simulink model "databydata"  (R2024a)
settings: Solver=FixedStepAuto  StartTime=0.0  StopTime=1  FixedStep=0.01  RelTol=1e-3
libraries: simulink x1
settings Model: Creator=wsl  LastModifiedBy=wsl

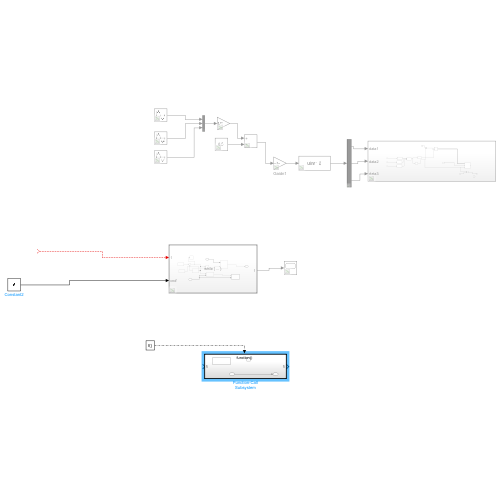
[thumbnail: Simulink's stored preview of the top-level diagram]
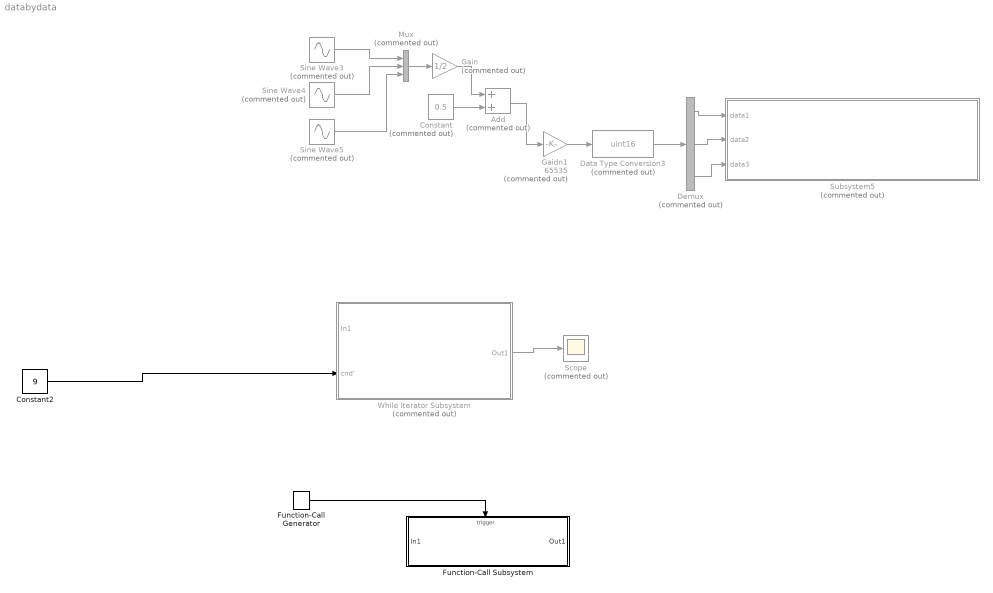
== system databydata ==
  Add : Sum  Commented=on
  Constant : Constant  Commented=on  Value=0.5
  Constant2 : Constant  Value=9
  Data Type Conversion3 : DataTypeConversion  Commented=on  OutDataTypeStr=uint16  SaturateOnIntegerOverflow=off  RndMeth=Floor
  Demux : Demux  Commented=on  Outputs=3
  Function-Call Generator : simulink/Ports & Subsystems/Function-Call Generator  sample_time=10  numberOfIterations=1  DisallowWideOutput=off
  Function-Call Subsystem : Subsystem  TreatAsAtomicUnit=on
  Gaidn1 : Gain  Commented=on  Gain=65535  ParamDataTypeStr=uint16
  Gain : Gain  Commented=on  Gain=1/2
  Mux : Mux  Commented=on  Inputs=3
  Scope : Scope  Commented=on
  Sine Wave3 : Sin  Commented=on  SineType=Sample based  SampleTime=0.0001
  Sine Wave4 : Sin  Commented=on  SineType=Sample based  SampleTime=0.0001  Offset=3
  Sine Wave5 : Sin  Commented=on  SineType=Sample based  SampleTime=0.0001  Offset=7
  Subsystem5 : Subsystem  Commented=on
  While Iterator Subsystem : Subsystem  Commented=on  TreatAsAtomicUnit=on
  wires:
  Gain/1 -> Add/1
  Add/1 -> Gaidn1/1
  Demux/2 -> Subsystem5/2(data2)
  Sine Wave3/1 -> Mux/1
  Demux/1 -> Subsystem5/1(data1)
  Sine Wave5/1 -> Mux/3
  Constant/1 -> Add/2
  Sine Wave4/1 -> Mux/2
  Gaidn1/1 -> Data Type Conversion3/1
  Data Type Conversion3/1 -> Demux/1
  Mux/1 -> Gain/1
  Demux/3 -> Subsystem5/3(data3)
  ? -> While Iterator Subsystem/1(In1)
  Constant2/1 -> While Iterator Subsystem/2(cnd')
  While Iterator Subsystem/1(Out1) -> Scope/1
  Function-Call Generator/1 -> Function-Call Subsystem/Trigger

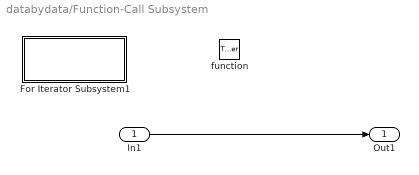
== system databydata/Function-Call Subsystem ==
  In1 : Inport
  function : TriggerPort  TriggerType=function-call  VariantControl=(inherit)
  For Iterator Subsystem1 : Subsystem  TreatAsAtomicUnit=on
  Out1 : Outport
  wires:
  In1/1 -> Out1/1

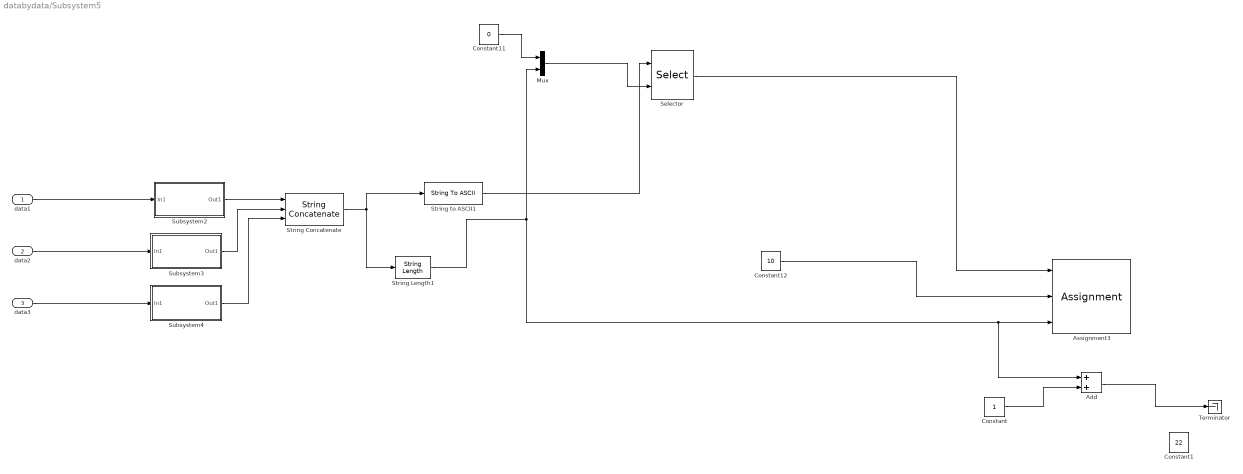
== system databydata/Subsystem5 ==
  data1 : Inport
  data2 : Inport  Port=2
  data3 : Inport  Port=3
  Add : Sum
  Assignment3 : Assignment  IndexMode=Zero-based  DiagnosticForDimensions=Warning  IndexOptions=Index vector (port)  Indices=2  OutputSizes=1
  Constant : Constant  OutDataTypeStr=uint8
  Constant1 : Constant  Value=22  OutDataTypeStr=uint8
  Constant11 : Constant  Value=0  OutDataTypeStr=uint8
  Constant12 : Constant  Value=10  OutDataTypeStr=uint8
  Mux : Mux  Inputs=2
  Selector : Selector  IndexMode=Zero-based  InputPortWidth=32  IndexOptions=Starting and ending indices (port)  Indices=[1 3]  OutputSizes=1
  String Concatenate : StringConcatenate  Inputs=3
  String Length1 : StringLength  OutDataTypeStr=uint8
  String to ASCII1 : StringToASCII  OutputVectorSize=32
  Subsystem2 : Subsystem
  Subsystem3 : Subsystem
  Subsystem4 : Subsystem
  Terminator : Terminator
  wires:
  data2/1 -> Subsystem3/1(In1)
  Subsystem4/1(Out1) -> String Concatenate/3
  data1/1 -> Subsystem2/1(In1)
  data3/1 -> Subsystem4/1(In1)
  Constant12/1 -> Assignment3/2
  String Length1/1 -> Add/1, Assignment3/3, Mux/2
  Subsystem3/1(Out1) -> String Concatenate/2
  Mux/1 -> Selector/2
  Subsystem2/1(Out1) -> String Concatenate/1
  Constant11/1 -> Mux/1
  String to ASCII1/1 -> Selector/1
  String Concatenate/1 -> String Length1/1, String to ASCII1/1
  Selector/1 -> Assignment3/1
  Constant/1 -> Add/2
  Add/1 -> Terminator/1

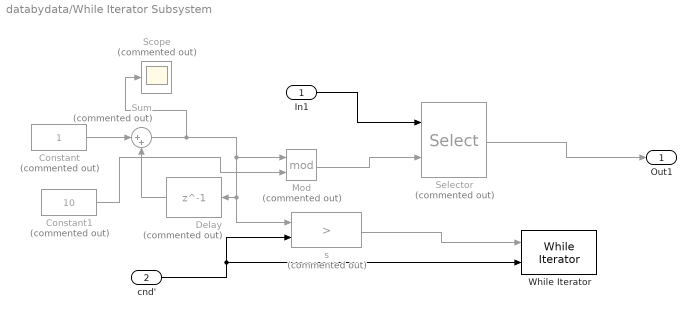
== system databydata/While Iterator Subsystem ==
  In1 : Inport
  cnd' : Inport  Port=2
  Constant : Constant  Commented=on
  Constant1 : Constant  Commented=on  Value=10
  Delay : Delay  Commented=on  DelayLength=1  InitialCondition=0  UseCircularBuffer=on
  Mod : Math  Commented=on  Operator=mod
  Scope : Scope  Commented=on
  Selector : Selector  Commented=on  IndexMode=Zero-based  InputPortWidth=9  IndexOptions=Index vector (port)  Indices=[1 3]  OutputSizes=1
  Sum : Sum  Commented=on  Inputs=|++
  While Iterator : WhileIterator  MaxIters=10
  s : RelationalOperator  Commented=on  Operator=>  OutDataTypeStr=boolean  InputSameDT=off
  Out1 : Outport
  wires:
  In1/1 -> Selector/1
  Constant/1 -> Sum/1
  Sum/1 -> Scope/1, Mod/1, s/1, Delay/1
  Delay/1 -> Sum/2
  s/1 -> While Iterator/1
  cnd'/1 -> While Iterator/2, s/2
  Selector/1 -> Out1/1
  Mod/1 -> Selector/2
  Constant1/1 -> Mod/2

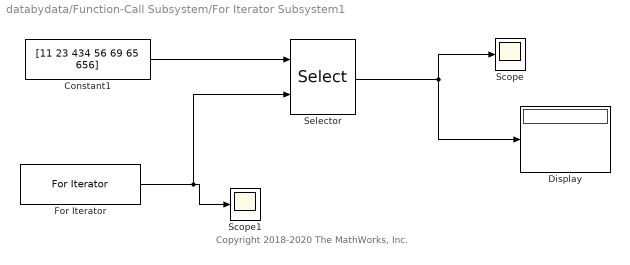
== system databydata/Function-Call Subsystem/For Iterator Subsystem1 ==
  note: Copyright 2018-2020 The MathWorks, Inc.
  Constant1 : Constant  Value=[11 23 434 56 69 65 656]
  Display : Display
  For Iterator : ForIterator  ResetStates=reset  IterationLimit=6  ExternalIncrement=on  IterationVariableDataType=double
  Scope : Scope
  Scope1 : Scope
  Selector : Selector  InputPortWidth=7  IndexOptions=Index vector (port)  Indices=[1 3]  OutputSizes=1
  wires:
  For Iterator/1 -> Scope1/1, Selector/2
  Constant1/1 -> Selector/1
  Selector/1 -> Display/1, Scope/1

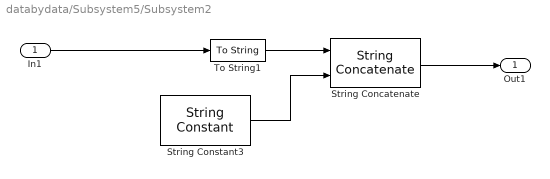
== system databydata/Subsystem5/Subsystem2 ==
  In1 : Inport
  String Concatenate : StringConcatenate
  String Constant3 : StringConstant  String="\",\""
  To String1 : ToString
  Out1 : Outport
  wires:
  To String1/1 -> String Concatenate/1
  String Concatenate/1 -> Out1/1
  In1/1 -> To String1/1
  String Constant3/1 -> String Concatenate/2

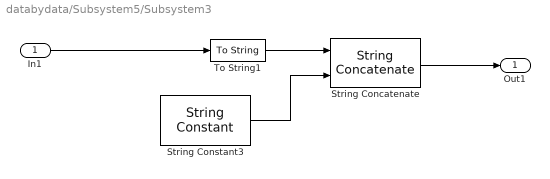
== system databydata/Subsystem5/Subsystem3 ==
  In1 : Inport
  String Concatenate : StringConcatenate
  String Constant3 : StringConstant  String="\",\""
  To String1 : ToString
  Out1 : Outport
  wires:
  To String1/1 -> String Concatenate/1
  String Concatenate/1 -> Out1/1
  In1/1 -> To String1/1
  String Constant3/1 -> String Concatenate/2

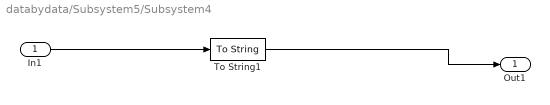
== system databydata/Subsystem5/Subsystem4 ==
  In1 : Inport
  To String1 : ToString
  Out1 : Outport
  wires:
  To String1/1 -> Out1/1
  In1/1 -> To String1/1
